simulink model "SVPWM_Base_MATLABfc1"  (R2020b)
settings: Solver=ode23tb  StartTime=0.0  StopTime=0.05  MaxStep=0.00001  RelTol=1e-3
libraries: simulink_extras x1, simulink x1
settings Model: Creator=15070  LastModifiedBy=15070

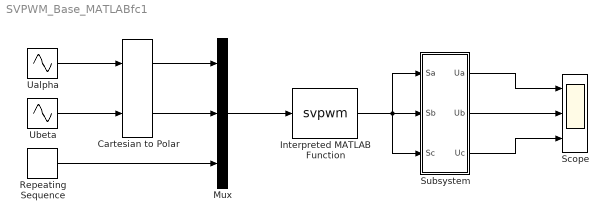
== system SVPWM_Base_MATLABfc1 ==
  Cartesian to Polar : simulink_extras/Transformations/Cartesian to Polar
  Interpreted MATLAB Function : MATLABFcn  MATLABFcn=svpwm
  Mux : Mux  Inputs=3
  Repeating Sequence : simulink/Sources/Repeating Sequence  rep_seq_t=[0 1/10000 1/5000]  rep_seq_y=[0 1/10000 0]
  Scope : Scope  NumInputPorts=3
  Subsystem : Subsystem  mask{Vdc=700}
  Ualpha : Sin  Amplitude=200  Frequency=2*50*pi  Phase=pi/2  SampleTime=10e-6
  Ubeta : Sin  Amplitude=200  Frequency=2*50*pi  SampleTime=10e-6
  wires:
  Ubeta/1 -> Cartesian to Polar/2
  Ualpha/1 -> Cartesian to Polar/1
  Repeating Sequence/1 -> Mux/3
  Cartesian to Polar/2 -> Mux/2
  Cartesian to Polar/1 -> Mux/1
  Mux/1 -> Interpreted MATLAB Function/1
  Interpreted MATLAB Function/1 -> Subsystem/1(Sa), Subsystem/3(Sc), Subsystem/2(Sb)
  Subsystem/2(Ub) -> Scope/2
  Subsystem/1(Ua) -> Scope/1
  Subsystem/3(Uc) -> Scope/3

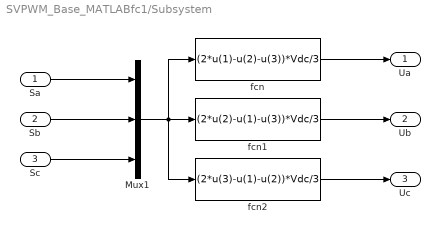
== system SVPWM_Base_MATLABfc1/Subsystem ==
  Sa : Inport
  Sb : Inport  Port=2
  Sc : Inport  Port=3
  Mux1 : Mux  Inputs=3
  fcn : Fcn  Expr=(2*u(1)-u(2)-u(3))*Vdc/3
  fcn1 : Fcn  Expr=(2*u(2)-u(1)-u(3))*Vdc/3
  fcn2 : Fcn  Expr=(2*u(3)-u(1)-u(2))*Vdc/3
  Ua : Outport
  Ub : Outport  Port=2
  Uc : Outport  Port=3
  wires:
  fcn2/1 -> Uc/1
  fcn1/1 -> Ub/1
  Sa/1 -> Mux1/1
  Sb/1 -> Mux1/2
  Mux1/1 -> fcn2/1, fcn1/1, fcn/1
  Sc/1 -> Mux1/3
  fcn/1 -> Ua/1
